simulink model "Model_1_AMBD"  (R2025b)
settings: Solver=VariableStepAuto  StartTime=0.0  StopTime=25  RelTol=1e-3
libraries: autolibshared x3
(part 1 of 3)
settings Model: Creator=HP  LastModifiedBy=HP

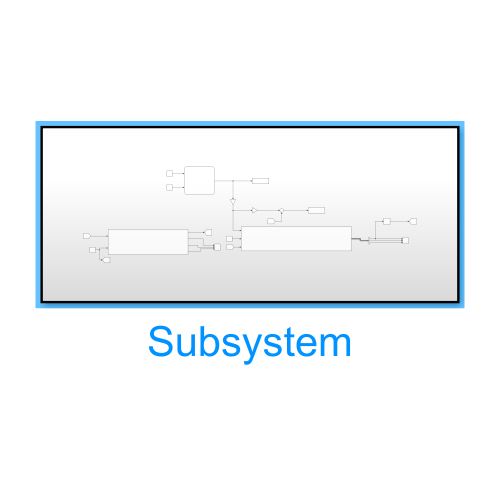
[thumbnail: Simulink's stored preview of the top-level diagram]
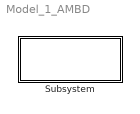
== system Model_1_AMBD ==
  Subsystem : Subsystem

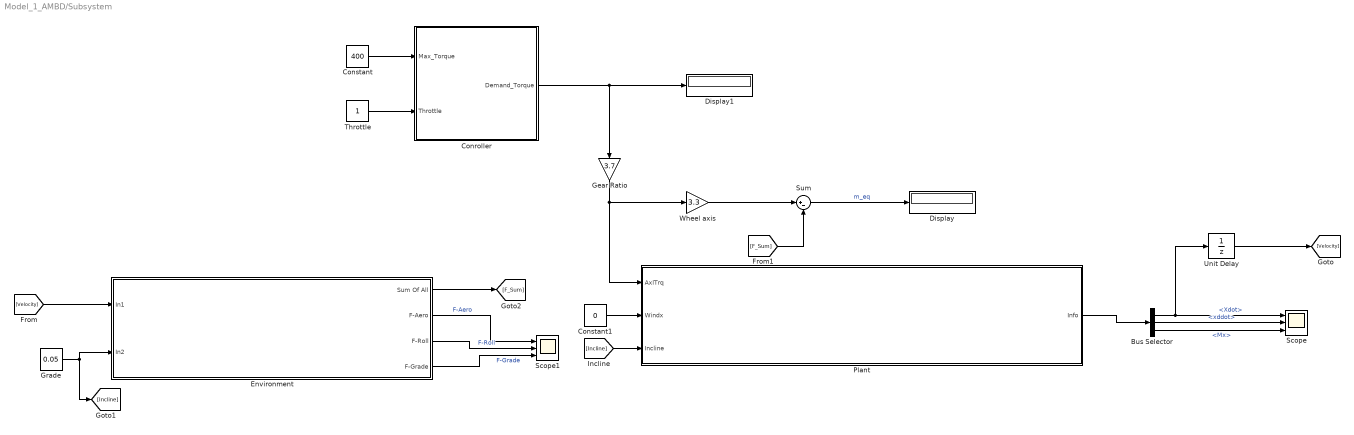
== system Model_1_AMBD/Subsystem ==
  Bus Selector : BusSelector  OutputSignals=InertFrm.Cg.Vel.Xdot,BdyFrm.Cg.Acc.xddot,BdyFrm.Moments.Drag.Mx
  Conroller : Stateflow chart  TreatAsAtomicUnit=on
  Constant : Constant  Value=400
  Constant1 : Constant  Value=0
  Display : Display
  Display1 : Display
  Environment : Subsystem
  Gear Ratio : Gain  Gain=3.7
  Grade : Constant  Value=0.05
  Plant : Subsystem
  Scope : Scope  NumInputPorts=3
      settings: ActiveDisplayYMinimum=-26.58392493787278  ActiveDisplayYMaximum=34.885049587543932
  Scope1 : Scope  NumInputPorts=3
      settings: ActiveDisplayYMinimum=-44.772246550179773  ActiveDisplayYMaximum=402.95021895161824
  Sum : Sum  Inputs=|+-
  Throttle : Constant
  Unit Delay : UnitDelay  SampleTime=-1  HasFrameUpgradeWarning=on
  Wheel axis : Gain  Gain=3.3
  wires:
  [Velocity] -> Environment/1(In1)
  Grade/1 -> Environment/2(In2), [Incline]
  Gear Ratio/1 -> Plant/1(AxlTrq), Wheel axis/1
  Plant/1(Info) -> Bus Selector/1
  Constant/1 -> Conroller/1(Max_Torque)
  Throttle/1 -> Conroller/2(Throttle)
  [Incline] -> Plant/3(Incline)
  Unit Delay/1 -> [Velocity]
  Bus Selector/3 -> Scope/3  "<Mx>"
  Bus Selector/2 -> Scope/2  "<xddot>"
  Bus Selector/1 -> Scope/1, Unit Delay/1  "<Xdot>"
  Constant1/1 -> Plant/2(Windx)
  Environment/2(F-Aero) -> Scope1/1  "F-Aero"
  Environment/3(F-Roll) -> Scope1/2  "F-Roll"
  Environment/4(F-Grade) -> Scope1/3  "F-Grade"
  Environment/1(Sum Of All) -> [F_Sum]
  Wheel axis/1 -> Sum/1
  [F_Sum] -> Sum/2
  Sum/1 -> Display/1  "m_eq"
  Conroller/1(Demand_Torque) -> Gear Ratio/1, Display1/1

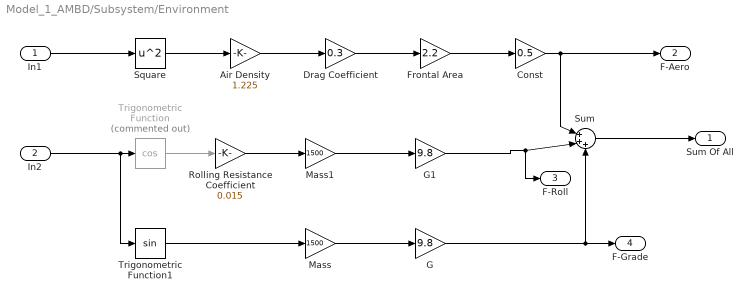
== system Model_1_AMBD/Subsystem/Environment ==
  In1 : Inport
  In2 : Inport  Port=2
  Air Density : Gain  Gain=1.225
  Const : Gain  Gain=0.5
  Drag Coefficient : Gain  Gain=0.3
  Frontal Area : Gain  Gain=2.2
  G : Gain  Gain=9.8
  G1 : Gain  Gain=9.8
  Mass : Gain  Gain=1500
  Mass1 : Gain  Gain=1500
  Rolling Resistance Coefficient : Gain  Gain=0.015
  Square : Math  Operator=square
  Sum : Sum  Inputs=|+++
  Trigonometric Function : Trigonometry  Commented=on  Operator=cos
  Trigonometric Function1 : Trigonometry
  Sum Of All : Outport
  F-Aero : Outport  Port=2
  F-Roll : Outport  Port=3
  F-Grade : Outport  Port=4
  wires:
  Trigonometric Function/1 -> Rolling Resistance Coefficient/1
  Trigonometric Function1/1 -> Mass/1
  Sum/1 -> Sum Of All/1
  Mass/1 -> G/1
  G/1 -> F-Grade/1, Sum/3
  Frontal Area/1 -> Const/1
  Mass1/1 -> G1/1
  Drag Coefficient/1 -> Frontal Area/1
  Const/1 -> F-Aero/1, Sum/1
  Rolling Resistance Coefficient/1 -> Mass1/1
  Square/1 -> Air Density/1
  Air Density/1 -> Drag Coefficient/1
  G1/1 -> F-Roll/1, Sum/2
  In2/1 -> Trigonometric Function1/1, Trigonometric Function/1
  In1/1 -> Square/1
